simulink model "Prob5_Simulink"  (R2022b)
settings: Solver=VariableStepAuto  StartTime=0.0  StopTime=tf  RelTol=1e-5
values from neighbouring files (symbols this model uses):
  A = [0 1 0 0 0 ... (first row only)    [Prob5_Elevator.m]
  B = [0 0 ... (first row only)    [Prob5_Elevator.m]
  C = [0 1 0 0 0 ... (first row only)    [Prob5_Elevator.m]
  D = [0 0 ... (first row only)    [Prob5_Elevator.m]
  ei = 15    [Prob5_Elevator.m]
  g = 9.81    [Prob5_Elevator.m]
  x0 = [0 0 0 0 0]'    [Prob5_Elevator.m]
settings Model: Creator=patlf  LastModifiedBy=patlf

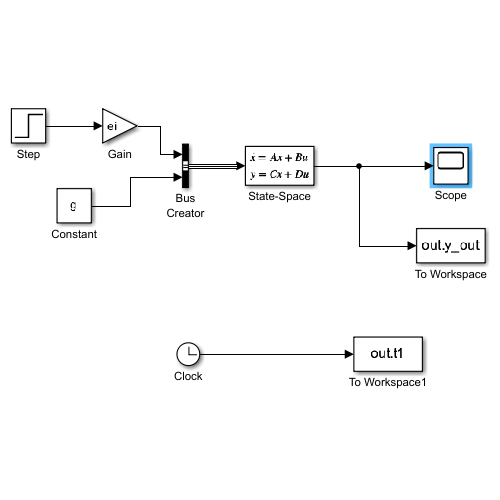
[thumbnail: Simulink's stored preview of the top-level diagram]
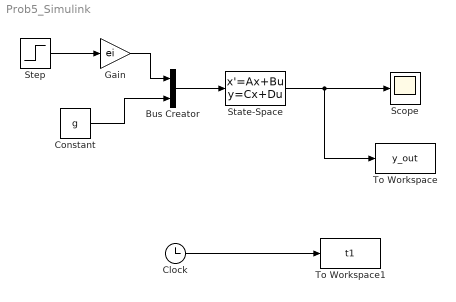
== system Prob5_Simulink ==
  Bus Creator : BusCreator  Inputs=2
  Clock : Clock
  Constant : Constant  Value=g
  Gain : Gain  Gain=ei
  Scope : Scope
  State-Space : StateSpace  A=A  B=B  C=C  D=D  InitialCondition=x0
  Step : Step  Time=0  SampleTime=0
  To Workspace : ToWorkspace  VariableName=y_out  SampleTime=-1
  To Workspace1 : ToWorkspace  VariableName=t1  SampleTime=-1
  wires:
  Step/1 -> Gain/1
  Constant/1 -> Bus Creator/2
  Gain/1 -> Bus Creator/1
  Bus Creator/1 -> State-Space/1
  State-Space/1 -> To Workspace/1, Scope/1
  Clock/1 -> To Workspace1/1
